simulink model "rl_sim_lin_compare"  (R2017a)
settings: Solver=FixedStepAuto  StartTime=0.0  StopTime=10  FixedStep=1/160000  RelTol=1e-3
undefined symbols (not defined in the file): H
libraries: dspmlti4 x2
settings Model: Creator=bhannigan  LastModifiedBy=bhannigan

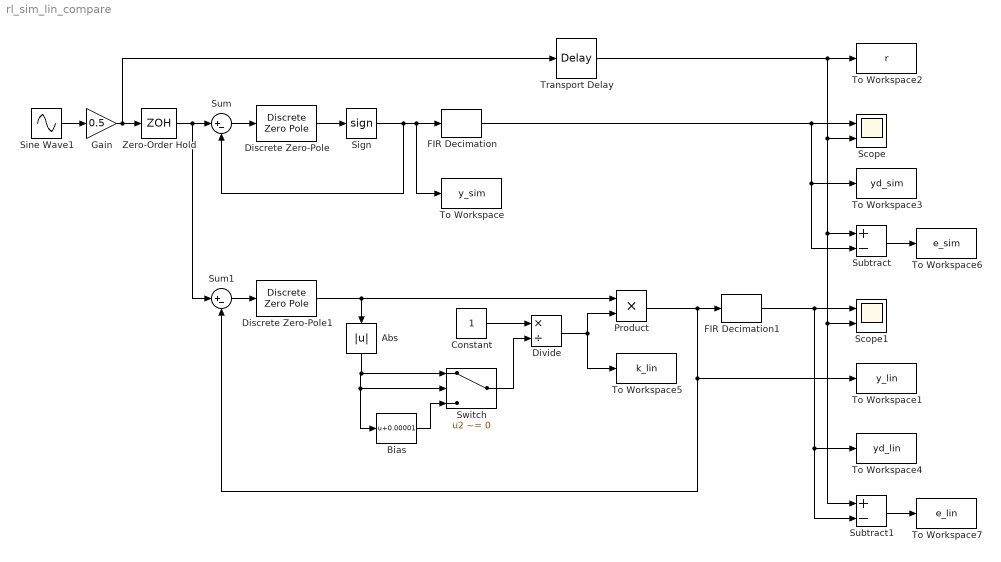
== system rl_sim_lin_compare ==
  Abs : Abs
  Bias : Bias  Bias=0.00001
  Constant : Constant
  Discrete Zero-Pole : DiscreteZeroPole  Zeros=H.Z{1}  Poles=H.P{1}  Gain=H.K  SampleTime=-1
  Discrete Zero-Pole1 : DiscreteZeroPole  Zeros=H.Z{1}  Poles=H.P{1}  Gain=H.K  SampleTime=-1
  Divide : Product  Inputs=*/
  FIR Decimation : dspmlti4/FIR Decimation  FilterSource=Dialog parameters  h=fir1(31,1/64)  D=32  filtStruct=Direct form  FilterObject=FDECIM  framing=Allow multirate processing  inputOffset=0  outputBufInitCond=0  roundingMode=Floor  overflowMode=off  firstCoeffDataTypeStr=Inherit: Same word length as input  firstCoeffMin=[]  firstCoeffMax=[]  firstCoeffLastDataTypeStr=Inherit: Same word length as input  outputDataTypeStr=Inherit: Same as accumulator  outputMin=[]  outputMax=[]  outputLastDataTypeStr=Inherit: Same as accumulator
  FIR Decimation1 : dspmlti4/FIR Decimation  FilterSource=Dialog parameters  h=fir1(31,1/64)  D=32  filtStruct=Direct form  FilterObject=FDECIM  framing=Allow multirate processing  inputOffset=0  outputBufInitCond=0  roundingMode=Floor  overflowMode=off  firstCoeffDataTypeStr=Inherit: Same word length as input  firstCoeffMin=[]  firstCoeffMax=[]  firstCoeffLastDataTypeStr=Inherit: Same word length as input  outputDataTypeStr=Inherit: Same as accumulator  outputMin=[]  outputMax=[]  outputLastDataTypeStr=Inherit: Same as accumulator
  Gain : Gain  Gain=0.5
  Product : Product
  Scope : Scope  NumInputPorts=2
  Scope1 : Scope  NumInputPorts=2
  Sign : Signum
  Sine Wave1 : Sin  Frequency=2*pi*20  SampleTime=0
  Subtract : Sum  Inputs=+-
  Subtract1 : Sum  Inputs=+-
  Sum : Sum  Inputs=|+-
  Sum1 : Sum  Inputs=|+-
  Switch : Switch  Criteria=u2 ~= 0
  To Workspace : ToWorkspace  VariableName=y_sim  SaveFormat=Timeseries  SampleTime=-1
  To Workspace1 : ToWorkspace  VariableName=y_lin  SaveFormat=Timeseries  SampleTime=-1
  To Workspace2 : ToWorkspace  VariableName=r  SaveFormat=Timeseries  SampleTime=-1
  To Workspace3 : ToWorkspace  VariableName=yd_sim  SaveFormat=Timeseries  SampleTime=-1
  To Workspace4 : ToWorkspace  VariableName=yd_lin  SaveFormat=Timeseries  SampleTime=-1
  To Workspace5 : ToWorkspace  VariableName=k_lin  SaveFormat=Timeseries  SampleTime=-1
  To Workspace6 : ToWorkspace  VariableName=e_sim  SaveFormat=Timeseries  SampleTime=-1
  To Workspace7 : ToWorkspace  VariableName=e_lin  SaveFormat=Timeseries  SampleTime=-1
  Transport Delay : TransportDelay  DelayTime=15/(32*200)
  Zero-Order Hold : ZeroOrderHold  SampleTime=1/(200*32)
  wires:
  Sum/1 -> Discrete Zero-Pole/1
  Discrete Zero-Pole/1 -> Sign/1
  Gain/1 -> Transport Delay/1, Zero-Order Hold/1
  Zero-Order Hold/1 -> Sum1/1, Sum/1
  Sign/1 -> Sum/2, To Workspace/1, FIR Decimation/1
  Sine Wave1/1 -> Gain/1
  FIR Decimation/1 -> Subtract/2, To Workspace3/1, Scope/1
  Discrete Zero-Pole1/1 -> Product/1, Abs/1
  Sum1/1 -> Discrete Zero-Pole1/1
  Constant/1 -> Divide/1
  Switch/1 -> Divide/2
  Product/1 -> FIR Decimation1/1, To Workspace1/1, Sum1/2
  FIR Decimation1/1 -> Subtract1/2, To Workspace4/1, Scope1/1
  Divide/1 -> Product/2, To Workspace5/1
  Abs/1 -> Switch/1, Switch/2, Bias/1
  Bias/1 -> Switch/3
  Transport Delay/1 -> Scope/2, Subtract/1, Subtract1/1, Scope1/2, To Workspace2/1
  Subtract/1 -> To Workspace6/1
  Subtract1/1 -> To Workspace7/1
